simulink model "compnesator_sim"  (R2017a)
settings: Solver=ode4  StartTime=0.0  StopTime=10  RelTol=1e-3
undefined symbols (not defined in the file or in its folder): sigbuilder_block
settings Model: Creator=Sean  LastModifiedBy=Sean

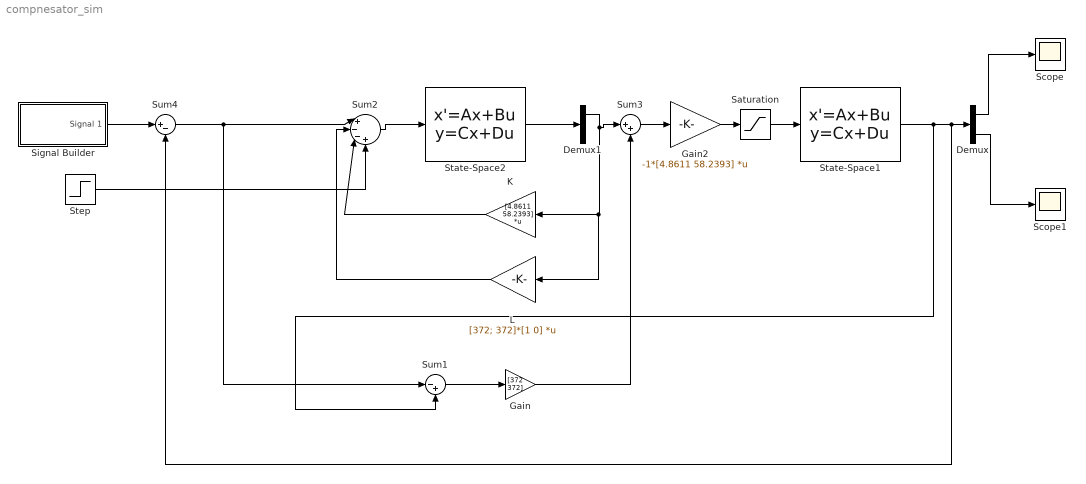
== system compnesator_sim ==
  Demux : Demux  Outputs=2
  Demux1 : Demux  Outputs=2
  Gain : Gain  Gain=[372 372]
  Gain2 : Gain  Gain=-1*[4.8611 58.2393]  Multiplication=Matrix(K*u)  SaturateOnIntegerOverflow=on
  K : Gain  Gain=[4.8611 58.2393]  Multiplication=Matrix(K*u)  SaturateOnIntegerOverflow=on
  L : Gain  Gain=[372; 372]*[1 0]  Multiplication=Matrix(K*u)
  Saturation : Saturate  UpperLimit=150  LowerLimit=-150
  Scope : Scope
  Scope1 : Scope
  Signal Builder : Subsystem  Tag=STV Subsys  LoadFcn=sigbuilder_block('load');  StartFcn=sigbuilder_block('start');  StopFcn=sigbuilder_block('stop');  ClipboardFcn=sigbuilder_block('clipboard');  mask(Sigbuilder block){tuvar=[0:10]}
      mask help: Simulink:masks:SigbuilderBlock_MD
      mask init:
      | if ~strcmp(get_param(bdroot(gcbh),'SimulationStatus'),'stopped') tuvar = sigbuilder_block('maskInit'); end
      settings: CopyFcn=sigbuilder_block('copy');  DeleteFcn=sigbuilder_block('delete');  ModelCloseFcn=sigbuilder_block('modelClose');  PreSaveFcn=sigbuilder_block('preSave');  PauseFcn=sigbuilder_block('pause');  ContinueFcn=sigbuilder_block('continue');  NameChangeFcn=sigbuilder_block('namechange');  OpenFcn=sigbuilder_block('open',[437.6 199.2 550.4 400 ]);  CloseFcn=sigbuilder_block('close');
      mask Display: plot(0, 0, 100, 100,[2, 2, 32, 32, 2], [68, 8, 8, 68, 68],[32, 2], [38, 38], [32, 19, 2],[53, 60, 44], [32, 17, 17, 2],[16, 16, 31, 31]);txt = getActiveGroup(gcbh);text(2, 100, txt,'verticalAlignment', 'top');
  State-Space1 : StateSpace  A=[0 10; 0 10]  B=[-0.55; 0.458]  C=eye(2)  D=[0; 0]  X0=0
  State-Space2 : StateSpace  A=[0 10; 0 10]  B=[-0.55; 0.458]  C=eye(2)  D=[0; 0]  X0=0
  Step : Step  SampleTime=0
  Sum1 : Sum  Inputs=|-+
  Sum2 : Sum  Inputs=|+--+  SaturateOnIntegerOverflow=on
  Sum3 : Sum  Inputs=|++
  Sum4 : Sum  Inputs=|+-
  wires:
  Gain2/1 -> Saturation/1
  State-Space1/1 -> Sum1/2, Sum4/2, Demux/1
  Demux/1 -> Scope/1
  Demux/2 -> Scope1/1
  Saturation/1 -> State-Space1/1
  K/1 -> Sum2/3
  L/1 -> Sum2/2
  Sum2/1 -> State-Space2/1
  Sum4/1 -> Sum2/1, Sum1/1
  Sum1/1 -> Gain/1
  Sum3/1 -> Gain2/1
  Gain/1 -> Sum3/2
  Signal Builder/1(Signal 1) -> Sum4/1
  State-Space2/1 -> Demux1/1
  Demux1/1 -> Sum3/1, L/1, K/1
  Step/1 -> Sum2/4

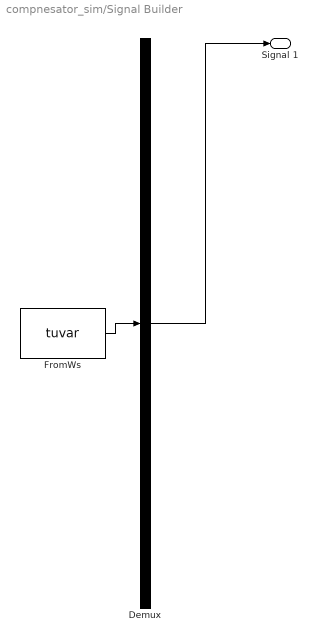
== system compnesator_sim/Signal Builder ==
  Demux : Demux  Tag=STV Demux  Outputs=1
  FromWs : FromWorkspace  Tag=STV FromWs  VariableName=tuvar  SampleTime=0
      SigBuilderData=|
      | common.afterFinalStr = 'Extrapolate'
      | common.sampleTime = 0
      | dataSet.timeRange = [0 10]
      | dataSet.name = 'Group 1'
      | sbobj.Groups.Name = 'Group 1'
      | sbobj.Groups.Signals.Name = 'Signal 1'
      | sbobj.Groups.Signals.XData = [0 3 3 10]
      | sbobj.Groups.Signals.YData = [1.5 1.5 -1.5 -1.5]
  Signal 1 : Outport  Tag=STV Outport
  wires:
  Demux/1 -> Signal 1/1
  FromWs/1 -> Demux/1
